simulink model "Comparacion"  (R2024a)
settings: Solver=VariableStepAuto  StartTime=0.0  StopTime=60  RelTol=1e-3
values from neighbouring files (symbols this model uses):
  betaF = 0.34*2*J_b    (= 9.52e-05)    [Linelizacion.m]
  den_G = [1 betaF/J (Lb*m_b+Lm*m_m)*g*cosd(theta_ref)/J]    [Linelizacion.m]
  g = 9.81    [Linelizacion.m]
  J = J_m + J_b    (= 0.0001400505562)    [Linelizacion.m]
  Kf = 0.001191    [Linelizacion.m]
  Lm = 0.135    [Linelizacion.m]
  m_m = 0.00339    [Linelizacion.m]
  num_G = (Lm/J)*Kf    (= 1.14804970692)    [Linelizacion.m]
undefined symbols (not defined in the file or in its folder): torqueB
libraries: simulink_extras x1, SignalEditorBlockLib x1
settings Model: Creator=alfar  LastModifiedBy=alfar

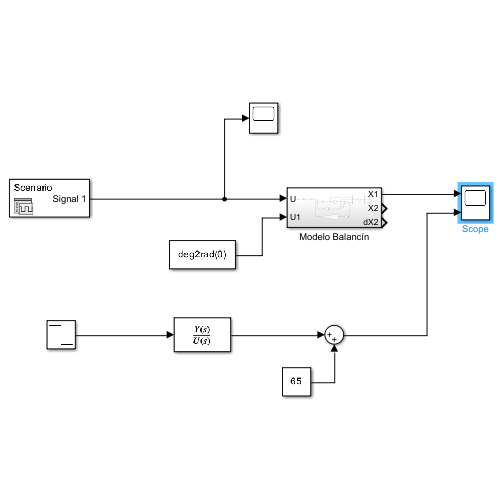
[thumbnail: Simulink's stored preview of the top-level diagram]
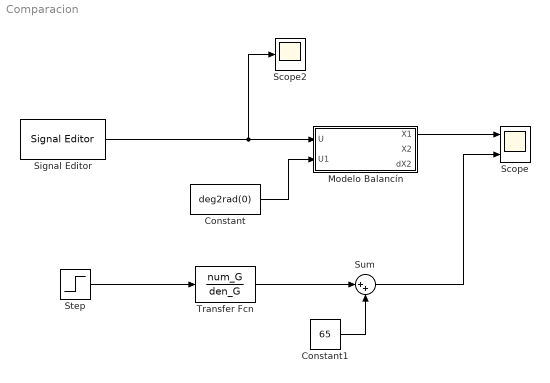
== system Comparacion ==
  Constant : Constant  Value=deg2rad(0)
  Constant1 : Constant  Value=65
  Modelo Balancín : Subsystem
  Scope : Scope  NumInputPorts=2
  Scope2 : Scope
  Signal Editor : SignalEditorBlockLib/Signal Editor  FileName=C:\Users\alfar\OneDrive\Escritorio\CONTROL\PROYECTO\Control-Aerobalancin\LINEALIZACION\TrenPulsos.mat  ActiveScenario=Scenario  ActiveSignal=Signal 1  IsBus=off  OutputBusObjectStr=Bus: BusObject  SampleTime=0  Interpolate=off  ZeroCross=off  OutputAfterFinalValue=Setting to zero  Unit=inherit  PreserveSignalName=on  ApplySigPropsToAllScenarios=on  ApplySigPropsToAllSignals=off
  Step : Step  Time=50  After=-5  SampleTime=0
  Sum : Sum  Inputs=|++
  Transfer Fcn : TransferFcn  Numerator=num_G  Denominator=den_G
  wires:
  Modelo Balancín/1(X1) -> Scope/1
  Constant/1 -> Modelo Balancín/2(U1)
  Transfer Fcn/1 -> Sum/1
  Signal Editor/1 -> Scope2/1, Modelo Balancín/1(U)
  Constant1/1 -> Sum/2
  Sum/1 -> Scope/2
  Step/1 -> Transfer Fcn/1

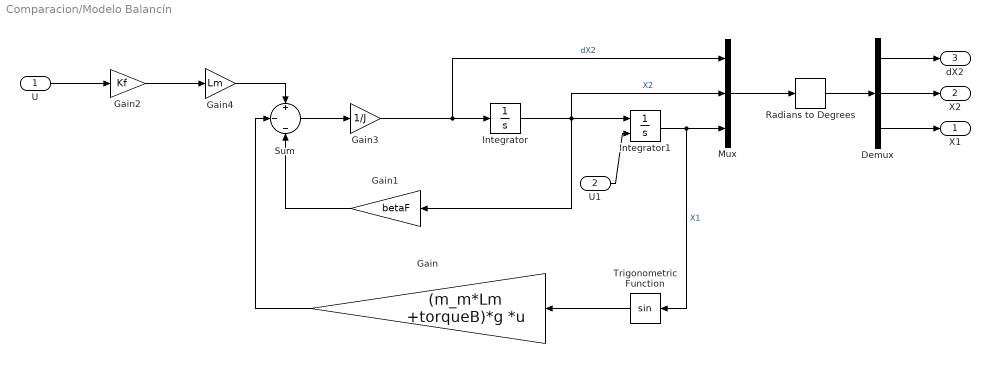
== system Comparacion/Modelo Balancín ==
  U : Inport
  U1 : Inport  Port=2
  Demux : Demux  Outputs=3
  Gain : Gain  Gain=(m_m*Lm +torqueB)*g  Multiplication=Matrix(K*u)
  Gain1 : Gain  Gain=betaF
  Gain2 : Gain  Gain=Kf
  Gain3 : Gain  Gain=1/J
  Gain4 : Gain  Gain=Lm
  Integrator : Integrator
  Integrator1 : Integrator  InitialConditionSource=external  InitialCondition=80*pi/180
  Mux : Mux  Inputs=3
  Radians to Degrees : simulink_extras/Transformations/Radians to Degrees
  Sum : Sum  Inputs=+|-|-
  Trigonometric Function : Trigonometry
  X1 : Outport
  X2 : Outport  Port=2
  dX2 : Outport  Port=3
  wires:
  Integrator/1 -> Mux/2, Integrator1/1, Gain1/1  "X2"
  Gain3/1 -> Mux/1, Integrator/1  "dX2"
  Trigonometric Function/1 -> Gain/1
  Mux/1 -> Radians to Degrees/1
  Gain/1 -> Sum/2
  Radians to Degrees/1 -> Demux/1
  Sum/1 -> Gain3/1
  Gain1/1 -> Sum/3
  Gain2/1 -> Gain4/1
  Integrator1/1 -> Mux/3, Trigonometric Function/1  "X1"
  U/1 -> Gain2/1
  U1/1 -> Integrator1/2
  Demux/1 -> dX2/1
  Demux/2 -> X2/1
  Demux/3 -> X1/1
  Gain4/1 -> Sum/1
